simulink model "Demo_original"  (R2025b)
settings: Solver=VariableStepAuto  StartTime=0.01  StopTime=6000  RelTol=1e-3
InitFcn:
  | initDemo
values from neighbouring files (symbols this model uses):
  dT = 0.01    [initDemo.m]
  x0 = [-15,12,deg2rad(90)]    [initDemo.m]
settings Model: Creator=kroni  LastModifiedBy=Space
settings SolverCC: AlgebraicLoopSolver=TrustRegion
settings DebuggingCC: UnconnectedInputMsg=warning  UnconnectedOutputMsg=warning  UnconnectedLineMsg=warning
settings ModelReferenceCC: EnableRefExpFcnMdlSchedulingChecks=on
settings RTWCC: GPUComputeCapability=3.5

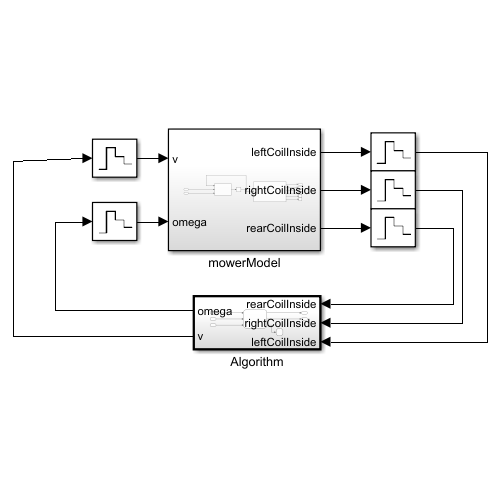
[thumbnail: Simulink's stored preview of the top-level diagram]
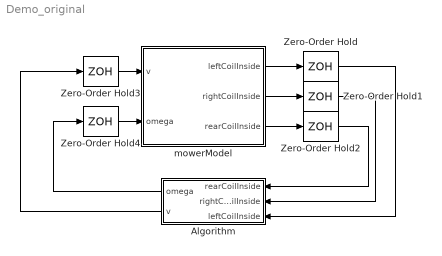
== system Demo_original ==
  Algorithm : Subsystem  TreatAsAtomicUnit=on  SystemSampleTime=dT
  Zero-Order Hold{,1..4} (5 alike) : ZeroOrderHold  SampleTime=dT
  mowerModel : Subsystem
  wires:
  Algorithm/2(v) -> Zero-Order Hold3/1
  Algorithm/1(omega) -> Zero-Order Hold4/1
  mowerModel/1(leftCoilInside) -> Zero-Order Hold/1
  mowerModel/2(rightCoilInside) -> Zero-Order Hold1/1
  Zero-Order Hold/1 -> Algorithm/3(leftCoilInside)
  Zero-Order Hold1/1 -> Algorithm/2(rightCoilInside)
  mowerModel/3(rearCoilInside) -> Zero-Order Hold2/1
  Zero-Order Hold2/1 -> Algorithm/1(rearCoilInside)
  Zero-Order Hold3/1 -> mowerModel/1(v)
  Zero-Order Hold4/1 -> mowerModel/2(omega)

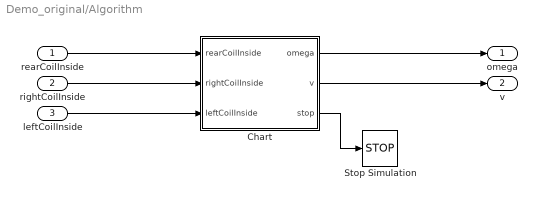
== system Demo_original/Algorithm ==
  rearCoilInside : Inport
  rightCoilInside : Inport  Port=2
  leftCoilInside : Inport  Port=3
  Chart : Stateflow chart  TreatAsAtomicUnit=on
  Stop Simulation : Stop
  omega : Outport
  v : Outport  Port=2
  wires:
  rightCoilInside/1 -> Chart/2(rightCoilInside)
  leftCoilInside/1 -> Chart/3(leftCoilInside)
  Chart/1(omega) -> omega/1
  Chart/2(v) -> v/1
  Chart/3(stop) -> Stop Simulation/1
  rearCoilInside/1 -> Chart/1(rearCoilInside)

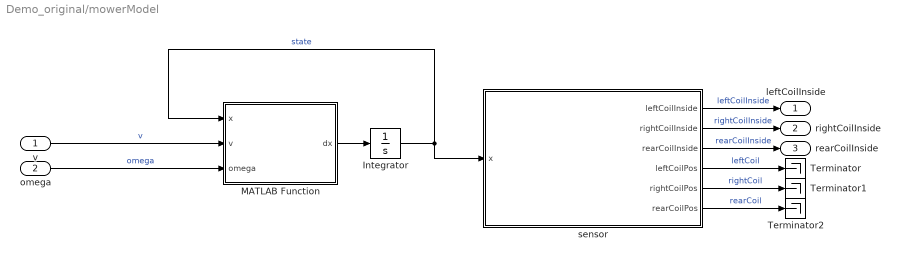
== system Demo_original/mowerModel ==
  v : Inport
  omega : Inport  Port=2
  Integrator : Integrator  InitialCondition=x0
  MATLAB Function : MATLAB Function  TreatAsAtomicUnit=on
  Terminator : Terminator
  Terminator1 : Terminator
  Terminator2 : Terminator
  sensor : MATLAB Function  TreatAsAtomicUnit=on
  leftCoilInside : Outport
  rightCoilInside : Outport  Port=2
  rearCoilInside : Outport  Port=3
  wires:
  Integrator/1 -> sensor/1(x), MATLAB Function/1(x)  "state"
  sensor/2(rightCoilInside) -> rightCoilInside/1  "rightCoilInside"
  omega/1 -> MATLAB Function/3(omega)  "omega"
  sensor/1(leftCoilInside) -> leftCoilInside/1  "leftCoilInside"
  MATLAB Function/1(dx) -> Integrator/1
  v/1 -> MATLAB Function/2(v)  "v"
  sensor/4(leftCoilPos) -> Terminator/1  "leftCoil"
  sensor/5(rightCoilPos) -> Terminator1/1  "rightCoil"
  sensor/3(rearCoilInside) -> rearCoilInside/1  "rearCoilInside"
  sensor/6(rearCoilPos) -> Terminator2/1  "rearCoil"

== matlab function Demo_original/mowerModel/sensor ==
  data: x input; leftCoilInside output; rightCoilInside output; rearCoilInside output; leftCoilPos output; rightCoilPos output; rearCoilPos output; gardenGeometry parameter
function [leftCoilInside, rightCoilInside,rearCoilInside,leftCoilPos,rightCoilPos,rearCoilPos] = sensor_model(x, gardenGeometry)

% initial conditions
leftCoilInside = false;
rightCoilInside = false;
rearCoilInside = false;

% lever arms
l1 = 0.5;
l2 = 0.2;
l3 = -0.05;

% coil position by transformation
leftCoilPos = [x(1)+l1*cos(x(3))-l2*sin(x(3)),x(2)+l1*sin(x(3))+l2*cos(x(3))];
rightCoilPos = [x(1)+l1*cos(x(3))+l2*sin(x(3)),x(2)+l1*sin(x(3))-l2*cos(x(3))];
rearCoilPos = [x(1)+l3*cos(x(3)),x(2)+l3*sin(x(3))];

% set inside / outside as virtual sensor
if inpolygon(leftCoilPos(1),leftCoilPos(2),gardenGeometry(:,1),gardenGeometry(:,2))
    leftCoilInside = true;
end
if inpolygon(rightCoilPos(1),rightCoilPos(2),gardenGeometry(:,1),gardenGeometry(:,2))
    rightCoilInside = true;
end
if inpolygon(rearCoilPos(1),rearCoilPos(2),gardenGeometry(:,1),gardenGeometry(:,2))
    rearCoilInside = true;
end

== matlab function Demo_original/mowerModel/MATLAB Function ==
  data: x input size=3; dx output size=3; v input; omega input
function dx = mower(x,v,omega)
% x = [x,y,psi]
    
    dx = zeros(3,1);

    dx(1) = v * cos(x(3)); 
    dx(2) = v * sin(x(3));
    dx(3) = omega;
end

== stateflow chart Demo_original/Algorithm/Chart ==
  state INIT
    en:
    stop = 0;
    du:
    v = 0;
    omega = 0;
  state DRIVE
    du:
    v = 0.5;
    omega = 0;
    ex:
    v = 0;
  state TURN_INSIDE
    du:
    v = 0;
    omega = 1;
  state TURNING
    du:
    omega = 1;
    v=0;
    ex:
    omega = 0;
    v = 0;
  state STOP
    du:
    v = 0;
    omega = 0;
    stop = 1;
  (default) -> INIT
  INIT -> TURN_INSIDE [order 2] : [leftCoilInside*rightCoilInside == 0]
  INIT -> STOP [order 3] : [~leftCoilInside*~rightCoilInside*~rearCoilInside == 0]
  INIT -> DRIVE [order 1] : [leftCoilInside == 1 & rightCoilInside == 1]
  DRIVE -> TURN_INSIDE [order 1] : [leftCoilInside*rightCoilInside == 0]
  TURNING -> DRIVE : [after(1+1.5*rand,sec)]
  TURN_INSIDE -> TURNING [order 2] : [leftCoilInside == 1 & rightCoilInside == 1]
  DRIVE -> STOP [order 2] : [~leftCoilInside*~rightCoilInside*~rearCoilInside == 1 & after(1,sec)]
  TURN_INSIDE -> STOP [order 1] : [~leftCoilInside*~rightCoilInside*~rearCoilInside == 1 & after(1,sec)]
  data: rearCoilInside input; rightCoilInside input; leftCoilInside input; omega output; v output; stop output
